simulink model "lab3_e2"  (R2016a)
settings: Solver=VariableStepAuto  StartTime=0.0  StopTime=500  RelTol=1e-3
values from neighbouring files (symbols this model uses):
  C_D = H'    [lab3_sumup.m]
  G_D = G'    [lab3_sumup.m]
  Gcl = dcgain(sys5)    [lab3_sumup.m]
  H_D = C'    [lab3_sumup.m]
  L_ndb = acker(G_D, H_D, [p0, p1])    [lab3_sumup.m]
  Ts = 0.75    [lab3_sumup.m]
libraries: simulink x1
settings Model: Creator=Helvins  LastModifiedBy=Helvins

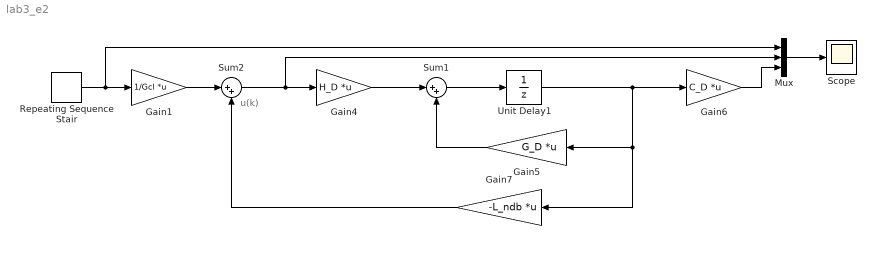
== system lab3_e2 ==
  note: u(k)
  Gain1 : Gain  Gain=1/Gcl  Multiplication=Matrix(K*u)
  Gain4 : Gain  Gain=H_D  Multiplication=Matrix(K*u)
  Gain5 : Gain  Gain=G_D  Multiplication=Matrix(K*u)
  Gain6 : Gain  Gain=C_D  Multiplication=Matrix(K*u)
  Gain7 : Gain  Gain=-L_ndb  Multiplication=Matrix(K*u)
  Mux : Mux  Inputs=3
  Repeating Sequence Stair : simulink/Sources/Repeating Sequence Stair  OutValues=[0, 0.7, -0.2, 0.5, 0].'  tsamp=200*Ts  OutMin=[]  OutMax=[]  OutDataTypeStr=double  OutputDataTypeScalingMode=double  OutDataType=fixdt(0,8)  ConRadixGroup=Best Precision: Vector-wise  OutScaling=2^-12
  Scope : Scope
  Sum1 : Sum  Inputs=|++
  Sum2 : Sum  Inputs=|++
  Unit Delay1 : UnitDelay  InitialCondition=[0; 0]  SampleTime=Ts
  wires:
  Gain4/1 -> Sum1/1
  Gain5/1 -> Sum1/2
  Sum1/1 -> Unit Delay1/1
  Unit Delay1/1 -> Gain5/1, Gain7/1, Gain6/1
  Gain7/1 -> Sum2/2
  Sum2/1 -> Mux/2, Gain4/1
  Gain1/1 -> Sum2/1
  Repeating Sequence Stair/1 -> Mux/1, Gain1/1
  Gain6/1 -> Mux/3
  Mux/1 -> Scope/1
